simulink model "INS"  (R2018a)
settings: Solver=FixedStepAuto  StartTime=0.0  StopTime=600  FixedStep=1/800  RelTol=1e-3
libraries: sharedutil x3, sharedtransform x3, simulink_extras x2, aerolibasang x1, sharedTrackingLibrary x1
settings Model: Creator=Daniel  LastModifiedBy=Daniel

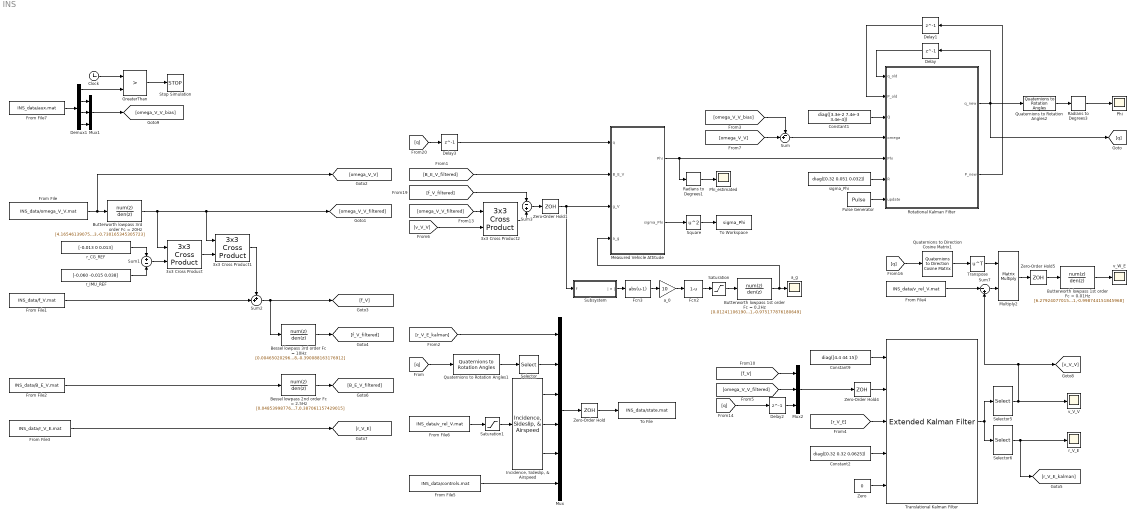
== system INS ==
  3x3 Cross Product : sharedutil/3x3 Cross Product  aMode=aMode
      settings: SourceProductBaseCode=AE
  3x3 Cross Product1 : sharedutil/3x3 Cross Product  aMode=aMode
      settings: SourceProductBaseCode=AE
  3x3 Cross Product2 : sharedutil/3x3 Cross Product  aMode=aMode
      settings: SourceProductBaseCode=AE
  Bessel lowpass 2nd order Fc = 2.5Hz : DiscreteFilter  Numerator=[0.048539987766887,0.097079975533774,0.048539987766887]  Denominator=[1,-1.192901206361467,0.387061157429015]
  Bessel lowpass 3rd order Fc = 10Hz : DiscreteFilter  Numerator=[0.004650202964924,0.013950608894772,0.013950608894772,0.004650202964924]  Denominator=[1,-2.135141627568843,1.562431414465148,-0.390088163176912]
  Butterworth lowpass 1st order Fc = 0.01Hz : DiscreteFilter  Numerator=[6.279240770159843e-04,6.279240770159843e-04]  Denominator=[1,-0.998744151845968]
  Butterworth lowpass 1st order Fc = 0.2Hz : DiscreteFilter  Numerator=[0.012411061909675,0.012411061909675]  Denominator=[1,-0.975177876180649]  InitialStates=1
  Butterworth lowpass 3rd order Fc = 20Hz : DiscreteFilter  Numerator=[4.165461390757476e-04,0.001249638417227,0.001249638417227,4.165461390757476e-04]  Denominator=[1,-2.686157396548144,2.419655110966473,-0.730165345305723]
  Clock : Clock
  Constant1 : Constant  Value=diag([3.3e-2 7.4e-3 3.4e-4])
  Constant2 : Constant  Value=diag([0.32 0.32 0.0625])
  Constant9 : Constant  Value=diag([4.4 44 15])
  Delay : Delay  DelayLength=1  InitialCondition=[1 0 0 0]  SampleTime=1/800
  Delay1 : Delay  DelayLength=1  InitialCondition=1e-2*eye(3)  SampleTime=1/800
  Delay2 : Delay  DelayLength=1  SampleTime=1/800
  Delay3 : Delay  DelayLength=1  InitialCondition=[1; 0; 0; 0]
  Demux1 : Demux
  Fcn2 : Fcn  Expr=1-u
  Fcn3 : Fcn  Expr=abs(u-1)
  From File : FromFile  FileName=INS_data/omega_V_V.mat  SampleTime=1/800  ExtrapolationBeforeFirstDataPoint=Ground value  InterpolationWithinTimeRange=Zero order hold  ExtrapolationAfterLastDataPoint=Ground value
  From File1 : FromFile  FileName=INS_data/f_V.mat  SampleTime=1/400  ExtrapolationBeforeFirstDataPoint=Ground value  InterpolationWithinTimeRange=Zero order hold  ExtrapolationAfterLastDataPoint=Ground value
  From File2 : FromFile  FileName=INS_data/B_E_V.mat  SampleTime=1/50  ExtrapolationBeforeFirstDataPoint=Ground value  InterpolationWithinTimeRange=Zero order hold  ExtrapolationAfterLastDataPoint=Ground value
  From File3 : FromFile  FileName=INS_data/r_V_E.mat  SampleTime=1/50  ExtrapolationBeforeFirstDataPoint=Ground value  InterpolationWithinTimeRange=Zero order hold  ExtrapolationAfterLastDataPoint=Ground value
  From File4 : FromFile  FileName=INS_data/v_rel_V.mat  SampleTime=1/50  ExtrapolationBeforeFirstDataPoint=Ground value  InterpolationWithinTimeRange=Zero order hold  ExtrapolationAfterLastDataPoint=Ground value
  From File5 : FromFile  FileName=INS_data/controls.mat  SampleTime=1/800  ExtrapolationBeforeFirstDataPoint=Ground value  InterpolationWithinTimeRange=Zero order hold  ExtrapolationAfterLastDataPoint=Ground value
  From File6 : FromFile  FileName=INS_data/v_rel_V.mat  SampleTime=1/50  ExtrapolationBeforeFirstDataPoint=Ground value  InterpolationWithinTimeRange=Zero order hold  ExtrapolationAfterLastDataPoint=Ground value
  From File7 : FromFile  FileName=INS_data/aux.mat  SampleTime=1/50  ExtrapolationBeforeFirstDataPoint=Ground value  InterpolationWithinTimeRange=Zero order hold  ExtrapolationAfterLastDataPoint=Ground value
  GreaterThan : RelationalOperator  Operator=>  OutDataTypeStr=boolean  RndMeth=Simplest
  "Incidence, Sideslip, & Airspeed" : aerolibasang/Incidence, Sideslip, & Airspeed
      settings: SourceProductName=Aerospace Blockset
  Measured Vehicle Attitude : MATLAB Function  TreatAsAtomicUnit=on
  Multiply2 : Product  Multiplication=Matrix(*)
  Mux : Mux  Inputs=6
  Mux1 : Mux  Inputs=3
  Mux2 : Mux  Inputs=3
  Phi : Scope
  Phi_estimated : Scope
  Pulse Generator : DiscretePulseGenerator  Period=16  PhaseDelay=15  SampleTime=1/800
  Quaternions to Direction Cosine Matrix1 : sharedtransform/Quaternions to  Direction Cosine Matrix  aMode=aMode
      settings: SourceProductName=Aerospace Blockset  SourceProductBaseCode=AE
  Quaternions to Rotation Angles1 : sharedtransform/Quaternions to Rotation Angles  rotationOrder=ZYX  aMode=aMode
      settings: SourceProductBaseCode=AE
  Quaternions to Rotation Angles2 : sharedtransform/Quaternions to Rotation Angles  rotationOrder=ZYX  aMode=aMode
      settings: SourceProductBaseCode=AE
  Radians to Degrees1 : simulink_extras/Transformations/Radians to Degrees
  Radians to Degrees3 : simulink_extras/Transformations/Radians to Degrees
  Rotational Kalman Filter : MATLAB Function  TreatAsAtomicUnit=on
  Saturation : Saturate  UpperLimit=1  LowerLimit=0
  Saturation1 : Saturate  UpperLimit=[inf inf inf]  LowerLimit=[0.1 -inf -inf]
  Selector : Selector  InputPortWidth=3  IndexOptions=Index vector (dialog)  Indices=[3 2 1]  OutputSizes=1
  Selector5 : Selector  InputPortWidth=6  IndexOptions=Index vector (dialog)  Indices=[1 2 3]  OutputSizes=1
  Selector6 : Selector  InputPortWidth=6  IndexOptions=Index vector (dialog)  Indices=[4 5 6]  OutputSizes=1
  Square : Math  Operator=square  SaturateOnIntegerOverflow=on
  Stop Simulation : Stop
  Subsystem : Subsystem
      mask Display:
      | disp("Calculate\nLoad Factor")
      | port_label('input', 1, '\bff', 'texmode', 'on')
      | port_label('output', 1, '\bf|n|', 'texmode', 'on')
  Sum : Sum  Inputs=-+|
  Sum1 : Sum  Inputs=+|-
  Sum2 : Sum  Inputs=++|
  Sum3 : Sum  Inputs=-|+
  Sum7 : Sum  Inputs=|-+
  To File : ToFile  Filename=INS_data/state.mat  MatrixName=state
  To Workspace : ToWorkspace  VariableName=sigma_Phi  SaveFormat=Timeseries  SampleTime=1/50
  Translational Kalman Filter : sharedTrackingLibrary/Extended Kalman Filter  StateTransitionFcn=kalman_trans_state  HasStateTransitionJacobianFcn=on  StateTransitionJacobianFcn=kalman_trans_state_jacobian  HasAdditiveProcessNoise=Nonadditive  ProcessNoise=1  HasTimeVaryingProcessNoise=on  HasStateTransitionFcnExtraArgument=1  InitialState=[0 0 0 0 0 0]  InitialStateCovariance=1e-1  MeasurementFcn1=kalman_trans_output  HasMeasurementJacobianFcn1=on  MeasurementJacobianFcn1=kalman_trans_output_jacobian  HasMeasurementEnablePort1=off  HasAdditiveMeasurementNoise1=Nonadditive  MeasurementNoise1=1  HasTimeVaryingMeasurementNoise1=on  HasMeasurementFcnExtraArgument1=1  MeasurementFcn2=myMeasurementFcn  HasMeasurementJacobianFcn2=off  HasMeasurementEnablePort2=off  HasAdditiveMeasurementNoise2=Additive  MeasurementNoise2=1  HasTimeVaryingMeasurementNoise2=off  HasMeasurementFcnExtraArgument2=0  MeasurementFcn3=myMeasurementFcn  HasMeasurementJacobianFcn3=off  HasMeasurementEnablePort3=off  HasAdditiveMeasurementNoise3=Additive  MeasurementNoise3=1  HasTimeVaryingMeasurementNoise3=off  HasMeasurementFcnExtraArgument3=0  MeasurementFcn4=myMeasurementFcn  HasMeasurementJacobianFcn4=off  HasMeasurementEnablePort4=off  HasAdditiveMeasurementNoise4=Additive  MeasurementNoise4=1  HasTimeVaryingMeasurementNoise4=off  HasMeasurementFcnExtraArgument4=0  MeasurementFcn5=myMeasurementFcn  HasMeasurementJacobianFcn5=off  HasMeasurementEnablePort5=off  HasAdditiveMeasurementNoise5=Additive  MeasurementNoise5=1  HasTimeVaryingMeasurementNoise5=off  HasMeasurementFcnExtraArgument5=0  EnableMultirate=on  StateTransitionFcnSampleTime=1/400  MeasurementFcn1SampleTime=1/50  MeasurementFcn2SampleTime=1  MeasurementFcn3SampleTime=1  MeasurementFcn4SampleTime=1  MeasurementFcn5SampleTime=1  UseCurrentEstimator=on  OutputStateCovariance=off  DataType=double  SampleTime=1/400  NumberOfMeasurements=1
      settings: SourceProductName=Control System Toolbox  SourceProductBaseCode=CT
  Transpose : Math  Operator=transpose  SaturateOnIntegerOverflow=on
  Zero : Constant  Value=0
  Zero-Order Hold : ZeroOrderHold  SampleTime=1/50
  Zero-Order Hold1 : ZeroOrderHold  SampleTime=1/50
  Zero-Order Hold4 : ZeroOrderHold  SampleTime=1/400
  Zero-Order Hold5 : ZeroOrderHold  SampleTime=1/50
  a_0 : Gain  Gain=10
  a_g : Scope
  r_CG_REF : Constant  Value=[-0.013 0 0.013]
  r_IMU_REF : Constant  Value=[-0.060 -0.015 0.038]
  r_V_E : Scope
  sigma_Phi : Constant  Value=diag([0.32 0.051 0.032])
  v_V_V : Scope
  v_W_E : Scope
  wires:
  From File/1 -> [omega_V_V], Butterworth lowpass 3rd order Fc = 20Hz/1
  r_CG_REF/1 -> Sum1/1
  r_IMU_REF/1 -> Sum1/2
  Sum1/1 -> 3x3 Cross Product/2
  3x3 Cross Product/1 -> 3x3 Cross Product1/2
  From File1/1 -> Sum2/2
  Butterworth lowpass 3rd order Fc = 20Hz/1 -> 3x3 Cross Product1/1, [omega_V_V_filtered], 3x3 Cross Product/1
  Mux2/1 -> Zero-Order Hold4/1
  Translational Kalman Filter/1 -> Selector5/1, Selector6/1
  Selector6/1 -> r_V_E/1, [r_V_E_kalman]
  [r_V_E] -> Translational Kalman Filter/3
  Zero-Order Hold4/1 -> Translational Kalman Filter/2
  From File4/1 -> Sum7/1
  Quaternions to Direction Cosine Matrix1/1 -> Transpose/1
  Transpose/1 -> Multiply2/1
  Sum7/1 -> Multiply2/2
  Multiply2/1 -> Zero-Order Hold5/1
  Quaternions to Rotation Angles2/1 -> Radians to Degrees3/1
  Radians to Degrees3/1 -> Phi/1
  Bessel lowpass 2nd order Fc = 2.5Hz/1 -> [B_E_V_filtered]
  From File2/1 -> Bessel lowpass 2nd order Fc = 2.5Hz/1
  [omega_V_V_filtered] -> Mux2/2
  [f_V] -> Mux2/1
  Bessel lowpass 3rd order Fc = 10Hz/1 -> [f_V_filtered]
  Sum2/1 -> Bessel lowpass 3rd order Fc = 10Hz/1, [f_V]
  [q] -> Delay2/1
  [q] -> Quaternions to Direction Cosine Matrix1/1
  Butterworth lowpass 1st order Fc = 0.01Hz/1 -> v_W_E/1
  Delay2/1 -> Mux2/3
  Zero-Order Hold5/1 -> Butterworth lowpass 1st order Fc = 0.01Hz/1
  Zero/1 -> Translational Kalman Filter/5
  Mux/1 -> Zero-Order Hold/1
  [q] -> Quaternions to Rotation Angles1/1
  Zero-Order Hold/1 -> To File/1
  From File6/1 -> Saturation1/1
  From File3/1 -> [r_V_E]
  [r_V_E_kalman] -> Mux/1
  Quaternions to Rotation Angles1/1 -> Selector/1
  "Incidence, Sideslip, & Airspeed"/1 -> Mux/3
  From File5/1 -> Mux/6
  Selector/1 -> Mux/2
  GreaterThan/1 -> Stop Simulation/1
  From File7/1 -> Demux1/1
  Demux1/2 -> Mux1/1
  Demux1/3 -> Mux1/2
  Demux1/4 -> Mux1/3
  Demux1/1 -> GreaterThan/2
  Clock/1 -> GreaterThan/1
  Mux1/1 -> [omega_V_V_bias]
  Constant2/1 -> Translational Kalman Filter/4
  Delay1/1 -> Rotational Kalman Filter/2(P_old)
  Delay/1 -> Rotational Kalman Filter/1(q_old)
  Rotational Kalman Filter/2(P_new) -> Delay1/1
  Rotational Kalman Filter/1(q_new) -> Quaternions to Rotation Angles2/1, [q], Delay/1
  Pulse Generator/1 -> Rotational Kalman Filter/7(update)
  Sum/1 -> Rotational Kalman Filter/4(omega)
  sigma_Phi/1 -> Rotational Kalman Filter/6(R)
  Fcn2/1 -> Saturation/1
  Constant1/1 -> Rotational Kalman Filter/3(Q)
  Saturation/1 -> Butterworth lowpass 1st order Fc = 0.2Hz/1
  Subsystem/1(| n |) -> Fcn3/1
  Fcn3/1 -> a_0/1
  a_0/1 -> Fcn2/1
  [omega_V_V_bias] -> Sum/1
  [omega_V_V] -> Sum/2
  [B_E_V_filtered] -> Measured Vehicle Attitude/2(B_E_V)
  [v_V_V] -> 3x3 Cross Product2/2
  [f_V_filtered] -> Sum3/1
  Sum3/1 -> Zero-Order Hold1/1
  3x3 Cross Product2/1 -> Sum3/2
  [omega_V_V_filtered] -> 3x3 Cross Product2/1
  Zero-Order Hold1/1 -> Subsystem/1(f), Measured Vehicle Attitude/3(g_V)
  Square/1 -> To Workspace/1
  Measured Vehicle Attitude/2(sigma_Phi) -> Square/1
  Radians to Degrees1/1 -> Phi_estimated/1
  Measured Vehicle Attitude/1(Phi) -> Rotational Kalman Filter/5(Phi), Radians to Degrees1/1
  [q] -> Delay3/1
  Delay3/1 -> Measured Vehicle Attitude/1(q)
  Selector5/1 -> v_V_V/1, Sum7/2, [v_V_V]
  Butterworth lowpass 1st order Fc = 0.2Hz/1 -> Measured Vehicle Attitude/4(a_g), a_g/1
  Constant9/1 -> Translational Kalman Filter/1
  "Incidence, Sideslip, & Airspeed"/2 -> Mux/4
  Saturation1/1 -> "Incidence, Sideslip, & Airspeed"/1
  "Incidence, Sideslip, & Airspeed"/3 -> Mux/5
  3x3 Cross Product1/1 -> Sum2/1

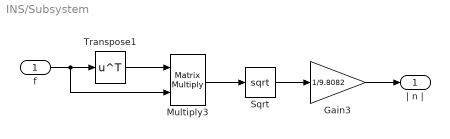
== system INS/Subsystem ==
  f : Inport
  Gain3 : Gain  Gain=1/9.8082
  Multiply3 : Product  Multiplication=Matrix(*)
  Sqrt : Sqrt  SaturateOnIntegerOverflow=on
  Transpose1 : Math  Operator=transpose  SaturateOnIntegerOverflow=on
  | n | : Outport
  wires:
  f/1 -> Transpose1/1, Multiply3/2
  Transpose1/1 -> Multiply3/1
  Sqrt/1 -> Gain3/1
  Multiply3/1 -> Sqrt/1
  Gain3/1 -> | n |/1

== matlab function INS/Measured Vehicle Attitude ==
  data: q input; B_E_V input; Phi output; g_V input; sigma_Phi output; a_g input
function [Phi, sigma_Phi] = fcn(q, B_E_V, g_V, a_g)

% Calculate earth base
B_E_E = [2.1048e-05; 1.5839e-06; 4.3789e-05];
g_E = [0; 0; 9.8082];

e1 = g_E/norm(g_E) + B_E_E/norm(B_E_E);
e1 = e1/norm(e1);

e2 = cross(g_E, B_E_E);
e2 = e2/norm(e2);

e3 = cross(e1, e2);

E = [e1 e2 e3];

% Calculate vehicle base
v1 = g_V/norm(g_V) + B_E_V/norm(B_E_V);
v1 = v1/norm(v1);

v2 = cross(g_V, B_E_V);
v2 = v2/norm(v2);

v3 = cross(v1, v2);

V = [v1 v2 v3];

% Get transformation matrix and pitch & bank
T_VE = V*E';

phi = atan2(T_VE(2,3), T_VE(3,3));
theta = -asin(T_VE(1,3));

% Compute yaw from magnetic field only
B_E_E = [2.1048e-05; 1.5839e-06; 4.3789e-05];

B_x = cos(theta)*B_E_V(1) + sin(phi)*sin(theta)*B_E_V(2) + cos(phi)*sin(theta)*B_E_V(3);
B_y = cos(phi)*B_E_V(2) - sin(phi)*B_E_V(3);

psi = atan2(B_E_E(2), B_E_E(1)) - atan2(B_y, B_x);
if psi > pi
    psi = psi - 2*pi;
end

% Get estimated yaw
psi_est = atan2(2*(q(2)*q(3) + q(1)*q(4)), q(1)^2 + q(2)^2 - q(3)^2 - q(4)^2);

% Blend estimated yaw and measured yaw together, via acceleration gain
delta_psi = psi - psi_est;

if delta_psi > pi
    delta_psi = delta_psi - 2*pi;
elseif delta_psi < -pi
    delta_psi = 2*pi + delta_psi;
end

psi = psi_est + a_g * delta_psi;

if psi > pi
    psi = psi - 2*pi;
elseif psi < -pi
    psi = 2*pi + psi;
end

Phi = [phi, theta, psi];

% Compute the standard deviations
sigma1 = [0.1102 0.3460 0.2041];
sigma2 = 4830.3*[sqrt(44*B_E_V(3)^2 + 4.7e-12*g_V(2)^2 + 15*B_E_V(2)^2 + 3.5e-12*g_V(3)^2);
                 sqrt(15*B_E_V(1)^2 + 1.5e-12*g_V(3)^2 + 4.4*B_E_V(3)^2 + 4.7e-12*g_V(1)^2);
                 sqrt(4.4*B_E_V(2)^2 + 3.5e-12*g_V(1)^2 + 44*B_E_V(1)^2 + 1.5e-12*g_V(2)^2)];
sigma3 = [sqrt(sigma1(2)^2*v2(3)^2 + sigma2(3)^2*v1(2)^2 + sigma1(3)^2*v2(2)^2 + sigma2(2)^2*v1(3)^2);
          sqrt(sigma1(3)^2*v2(1)^2 + sigma2(1)^2*v1(3)^2 + sigma1(1)^2*v2(3)^2 + sigma2(3)^2*v1(1)^2);
          sqrt(sigma1(1)^2*v2(2)^2 + sigma2(2)^2*v1(1)^2 + sigma1(2)^2*v2(1)^2 + sigma2(1)^2*v1(2)^2)];

sigma_13 = sqrt(e1(3)^2*sigma1(1)^2 + e2(3)^2*sigma2(1)^2 + e3(3)^2*sigma3(1)^2);
sigma_23 = sqrt(e1(3)^2*sigma1(2)^2 + e2(3)^2*sigma2(2)^2 + e3(3)^2*sigma3(2)^2);
sigma_33 = sqrt(e1(3)^2*sigma1(3)^2 + e2(3)^2*sigma2(3)^2 + e3(3)^2*sigma3(3)^2);
      
sigma_phi = 1/(T_VE(3,3)/T_VE(2,3) + T_VE(2,3)/T_VE(3,3))*sqrt((sigma_23/T_VE(2,3))^2 + (sigma_33/T_VE(3,3))^2);
sigma_theta = 1/sqrt(1 - T_VE(1,3)^2)*sigma_13;

sigma_Bx = sqrt(cos(theta)^2*1.5e-12 + (sin(phi)*sin(theta))^2*3.5e-12 + (cos(phi)*sin(theta))^2*4.7e-12 ...
                + (cos(phi)*sin(theta)*B_E_V(2) - sin(phi)*sin(theta)*B_E_V(3))^2*sigma_phi^2 ...
                + (sin(theta)*B_E_V(1) - sin(phi)*cos(theta)*B_E_V(2) - cos(phi)*cos(theta)*B_E_V(3))^2*sigma_theta^2);
sigma_By = sqrt(cos(phi)^2*3.5e-12 + sin(phi)^2*4.7e-12 + (sin(phi)*B_E_V(2) + cos(phi)*B_E_V(3))^2*sigma_phi^2);

sigma_psi = 1/(B_x/B_y + B_y/B_x)*sqrt((sigma_Bx/B_x)^2 + (sigma_By/B_y)^2);

sigma_Phi = [sigma_phi; sigma_theta; a_g*sigma_psi];

== matlab function INS/Rotational Kalman Filter ==
  data: q_old input; P_old input; q_new output; Q input; omega input; Phi input; R input; P_new output; update input
function [q_new, P_new] = fcn(q_old, P_old, Q, omega, Phi, R, update)
%% Predict (800Hz)
Ts = 1/800;

% Predict the new full quaternion state
F = [1             -Ts/2*omega(1) -Ts/2*omega(2) -Ts/2*omega(3);
     Ts/2*omega(1)  1              Ts/2*omega(3) -Ts/2*omega(2);
     Ts/2*omega(2) -Ts/2*omega(3)  1              Ts/2*omega(1);
     Ts/2*omega(3)  Ts/2*omega(2) -Ts/2*omega(1)  1];
 
q_new = F*q_old;
q_new = q_new / norm(q_new);

% Predict the new reduced state covariance matrix
F = [1            Ts*omega(3) -Ts*omega(2);
    -Ts*omega(3)  1            Ts*omega(1);
     Ts*omega(2) -Ts*omega(1)  1];

P_new = F*P_old*F' + Ts^2/4*Q;

%% Update (50Hz)
if update
    % Compute the measured quaternion from measured attitude
    phi = Phi(1);
    theta = Phi(2);
    psi = Phi(3);
    
    q = [cos(phi/2)*cos(theta/2)*cos(psi/2) + sin(phi/2)*sin(theta/2)*sin(psi/2);
         sin(phi/2)*cos(theta/2)*cos(psi/2) - cos(phi/2)*sin(theta/2)*sin(psi/2);
    	 cos(phi/2)*sin(theta/2)*cos(psi/2) + sin(phi/2)*cos(theta/2)*sin(psi/2);
    	 cos(phi/2)*cos(theta/2)*sin(psi/2) - sin(phi/2)*sin(theta/2)*cos(psi/2)];
    
     % Match the sign of the computed quaternion with estimated quaternion
    if sign(q(1)) ~= sign(q_new(1))
        q = -q;
    end
    
    % Compute the error quaternion
    J = [-q_new(2) -q_new(3) -q_new(4);
          q_new(1) -q_new(4)  q_new(3);
          q_new(4)  q_new(1) -q_new(2);
         -q_new(3)  q_new(2)  q_new(1)];
    
    delta_q = J'*q;
    
    % Compute the Kalman gain
    T11 = q_new(1)^2 + q_new(2)^2 - q_new(3)^2 - q_new(4)^2;
    T12 = 2*(q_new(2)*q_new(3) + q_new(1)*q_new(4));
    T13 = 2*(q_new(2)*q_new(4) - q_new(1)*q_new(3));
    T23 = 2*(q_new(3)*q_new(4) + q_new(1)*q_new(2));
    T33 = q_new(1)^2 - q_new(2)^2 - q_new(3)^2 + q_new(4)^2;
    
    phi_new = atan2(T23, T33);
    theta_new = -asin(T13);
    psi_new = atan2(T12, T11);
    
    r_ = [cos(phi_new/2)*cos(theta_new/2)*cos(psi_new/2) - sin(phi_new/2)*sin(theta_new/2)*sin(psi_new/2);
          sin(phi_new/2)*cos(theta_new/2)*cos(psi_new/2) + cos(phi_new/2)*sin(theta_new/2)*sin(psi_new/2);
          cos(phi_new/2)*sin(theta_new/2)*cos(psi_new/2) - sin(phi_new/2)*cos(theta_new/2)*sin(psi_new/2);
          cos(phi_new/2)*cos(theta_new/2)*sin(psi_new/2) + sin(phi_new/2)*sin(theta_new/2)*cos(psi_new/2)];
    
    q_ = [cos(phi_new/2)*cos(theta_new/2)*cos(psi_new/2) + sin(phi_new/2)*sin(theta_new/2)*sin(psi_new/2);
          sin(phi_new/2)*cos(theta_new/2)*cos(psi_new/2) - cos(phi_new/2)*sin(theta_new/2)*sin(psi_new/2);
          cos(phi_new/2)*sin(theta_new/2)*cos(psi_new/2) + sin(phi_new/2)*cos(theta_new/2)*sin(psi_new/2);
          cos(phi_new/2)*cos(theta_new/2)*sin(psi_new/2) - sin(phi_new/2)*sin(theta_new/2)*cos(psi_new/2)];
    
    L = 1/2*[-q_(2) -r_(3) -q_(4);
              q_(1) -r_(4) -q_(3);
              q_(4)  r_(1)  q_(2);
             -q_(3) -r_(2)  q_(1)];
    
    M = J'*L;
    
    K = P_new*(P_new + M*R*M')^(-1);
    
    % Update the reduced state vector and error covariance matrix
    delta_q = K*delta_q;
    P_new = (eye(3) - K)*P_new;
    
    % Update the full state vector
    q_new = q_new + J*delta_q;
    q_new = q_new/norm(q_new);
end
